simulink model "thumb_model_based_control"  (Simulink 6.6)
settings: Solver=ode45  StartTime=0.0  StopTime=10.0  RelTol=1e-3
libraries: simulink x3, dspmtrx3 x1
settings Model: Creator=Jadav Das  LastModifiedBy=Jadav Das

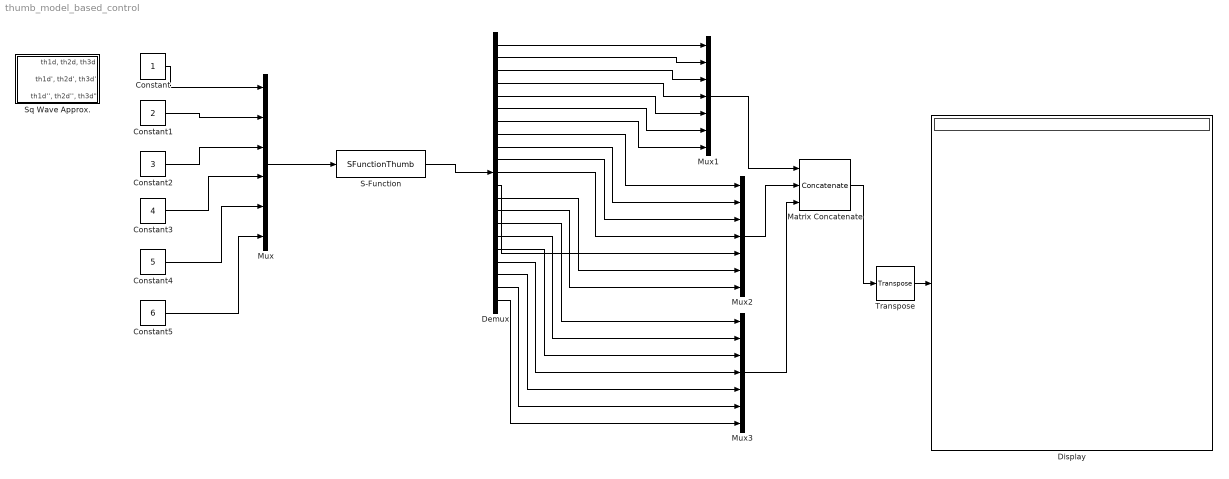
== system thumb_model_based_control ==
  Constant : Constant
  Constant1 : Constant  Value=2
  Constant2 : Constant  Value=3
  Constant3 : Constant  Value=4
  Constant4 : Constant  Value=5
  Constant5 : Constant  Value=6
  Demux : Demux  Outputs=21
  Display : Display
  Matrix Concatenate : Concatenate  NumInputs=3  Mode=Multidimensional array  ConcatenateDimension=2
  Mux : Mux  Inputs=6
  Mux1 : Mux  Inputs=7
  Mux2 : Mux  Inputs=7
  Mux3 : Mux  Inputs=7
  S-Function : S-Function  FunctionName=SFunctionThumb
  Sq Wave Approx. : Subsystem
  Transpose : dspmtrx3/Transpose  SystemSampleTime=-1  Hermitian=off  overflowFlag=off
  wires:
  Constant/1 -> Mux/1
  Constant1/1 -> Mux/2
  Constant2/1 -> Mux/3
  Constant3/1 -> Mux/4
  Constant4/1 -> Mux/5
  Constant5/1 -> Mux/6
  Mux/1 -> S-Function/1
  S-Function/1 -> Demux/1
  Demux/1 -> Mux1/1
  Demux/2 -> Mux1/2
  Demux/3 -> Mux1/3
  Demux/4 -> Mux1/4
  Demux/5 -> Mux1/5
  Demux/6 -> Mux1/6
  Demux/7 -> Mux1/7
  Demux/8 -> Mux2/1
  Demux/9 -> Mux2/2
  Demux/10 -> Mux2/3
  Demux/11 -> Mux2/4
  Demux/12 -> Mux2/5
  Demux/13 -> Mux2/6
  Demux/14 -> Mux2/7
  Demux/15 -> Mux3/1
  Demux/16 -> Mux3/2
  Demux/17 -> Mux3/3
  Demux/18 -> Mux3/4
  Demux/19 -> Mux3/5
  Demux/20 -> Mux3/6
  Demux/21 -> Mux3/7
  Mux1/1 -> Matrix Concatenate/1
  Mux2/1 -> Matrix Concatenate/2
  Mux3/1 -> Matrix Concatenate/3
  Matrix Concatenate/1 -> Transpose/1
  Transpose/1 -> Display/1

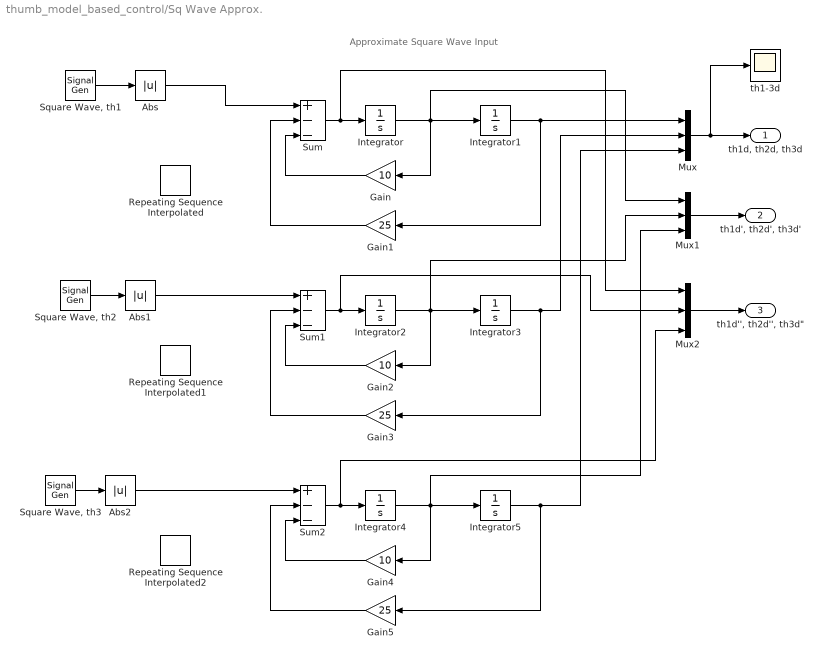
== system thumb_model_based_control/Sq Wave Approx. ==
  note: Approximate Square Wave Input
  Abs : Abs
  Abs1 : Abs
  Abs2 : Abs
  Gain : Gain  Orientation=left  Gain=10  SaturateOnIntegerOverflow=on
  Gain1 : Gain  Orientation=left  Gain=25  SaturateOnIntegerOverflow=on
  Gain2 : Gain  Orientation=left  Gain=10  SaturateOnIntegerOverflow=on
  Gain3 : Gain  Orientation=left  Gain=25  SaturateOnIntegerOverflow=on
  Gain4 : Gain  Orientation=left  Gain=10  SaturateOnIntegerOverflow=on
  Gain5 : Gain  Orientation=left  Gain=25  SaturateOnIntegerOverflow=on
  Integrator{,1..5} (6 alike) : Integrator
  Mux : Mux  Inputs=3
  Mux1 : Mux  Inputs=3
  Mux2 : Mux  Inputs=3
  Repeating Sequence Interpolated : simulink/Sources/Repeating Sequence Interpolated  SystemSampleTime=-1  OutValues=[0 90*pi/180 0 0].'  TimeValues=[0 1 2 3].'  LookUpMeth=Interpolation-Use End Values  tsamp=0.01  OutputDataTypeScalingMode=Specify via dialog  OutDataType=float('double')  OutScaling=2^-10
  Repeating Sequence Interpolated1 : simulink/Sources/Repeating Sequence Interpolated  SystemSampleTime=-1  OutValues=[0*pi/180 190*pi/180 45*pi/180 0*pi/180].'  TimeValues=[0 1 2 3].'  LookUpMeth=Interpolation-Use End Values  tsamp=0.01  OutputDataTypeScalingMode=Specify via dialog  OutDataType=float('double')  OutScaling=2^-10
  Repeating Sequence Interpolated2 : simulink/Sources/Repeating Sequence Interpolated  SystemSampleTime=-1  OutValues=[pi 90*pi/180 pi pi].'  TimeValues=[0 1 2 3].'  LookUpMeth=Interpolation-Use End Values  tsamp=0.01  OutputDataTypeScalingMode=Specify via dialog  OutDataType=float('double')  OutScaling=2^-10
  "Square Wave, th1" : SignalGenerator  Amplitude=10  Frequency=.2
  "Square Wave, th2" : SignalGenerator  Amplitude=10  Frequency=.2
  "Square Wave, th3" : SignalGenerator  Amplitude=10  Frequency=.2
  Sum : Sum  Inputs=+--  SaturateOnIntegerOverflow=on  InputSameDT=on
  Sum1 : Sum  Inputs=+--  SaturateOnIntegerOverflow=on  InputSameDT=on
  Sum2 : Sum  Inputs=+--  SaturateOnIntegerOverflow=on  InputSameDT=on
  th1-3d : Scope
  "th1d, th2d, th3d" : Outport
  "th1d', th2d', th3d'" : Outport  Port=2
  "th1d'', th2d'', th3d\"" : Outport  Port=3
  wires:
  Mux2/1 -> "th1d'', th2d'', th3d\""/1
  Mux1/1 -> "th1d', th2d', th3d'"/1
  Mux/1 -> "th1d, th2d, th3d"/1, th1-3d/1
  Sum1/1 -> Mux2/2, Integrator2/1
  Integrator3/1 -> Mux/2, Gain3/1
  Gain3/1 -> Sum1/2
  Gain2/1 -> Sum1/3
  Integrator2/1 -> Mux1/2, Gain2/1, Integrator3/1
  Sum/1 -> Mux2/1, Integrator/1
  Integrator1/1 -> Mux/1, Gain1/1
  Gain1/1 -> Sum/2
  Gain/1 -> Sum/3
  Integrator/1 -> Mux1/1, Gain/1, Integrator1/1
  Sum2/1 -> Integrator4/1, Mux2/3
  Integrator5/1 -> Gain5/1, Mux/3
  Gain5/1 -> Sum2/2
  Gain4/1 -> Sum2/3
  Integrator4/1 -> Integrator5/1, Gain4/1, Mux1/3
  "Square Wave, th1"/1 -> Abs/1
  "Square Wave, th2"/1 -> Abs1/1
  "Square Wave, th3"/1 -> Abs2/1
  Abs/1 -> Sum/1
  Abs1/1 -> Sum1/1
  Abs2/1 -> Sum2/1
